simulink model "LAB01P01_simulink"  (R2014a)
settings: Solver=ode45  StartTime=0.0  StopTime=Tstop  MaxStep=1e-5  MinStep=1e-6  RelTol=1e-3
values from neighbouring files (symbols this model uses):
  C1 = 1e-6    (= 1e-06)    [LAB01P01.m]
  C2 = 1e-6    (= 1e-06)    [LAB01P01.m]
  R1 = 1000    [LAB01P01.m]
  R2 = 1000    [LAB01P01.m]
  x0 = [0 0]    [LAB01P01.m]    (also in LAB01P03.m = [0 0]')
settings Model: Creator=S191436  LastModifiedBy=S191436

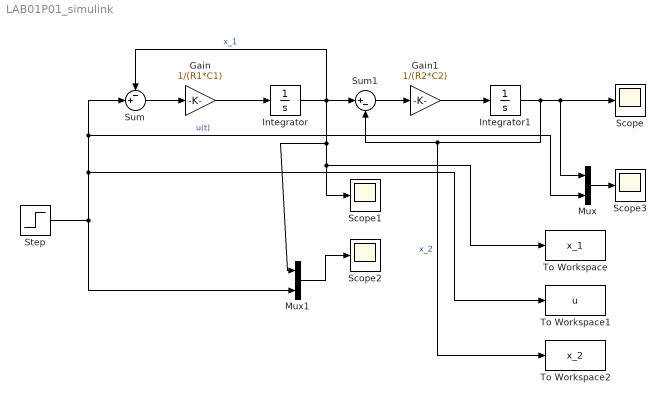
== system LAB01P01_simulink ==
  Gain : Gain  Gain=1/(R1*C1)
  Gain1 : Gain  Gain=1/(R2*C2)
  Integrator : Integrator  InitialCondition=x0(1)
  Integrator1 : Integrator  InitialCondition=x0(2)
  Mux : Mux  Inputs=2
  Mux1 : Mux  Inputs=2
  Scope{,1..3} (4 alike) : Scope
      Scope2 settings: SaveName=ScopeData2
      Scope3 settings: SaveName=ScopeData3
  Step : Step  Time=0  After=2  SampleTime=0
  Sum : Sum  Inputs=-+|
  Sum1 : Sum  Inputs=|+-
  To Workspace : ToWorkspace  VariableName=x_1  SaveFormat=Timeseries  SampleTime=-1
  To Workspace1 : ToWorkspace  VariableName=u  SaveFormat=Timeseries  SampleTime=-1
  To Workspace2 : ToWorkspace  VariableName=x_2  SaveFormat=Timeseries  SampleTime=-1
  wires:
  Gain1/1 -> Integrator1/1
  Sum1/1 -> Gain1/1
  Integrator/1 -> Mux1/1, To Workspace/1, Scope1/1, Sum1/1, Sum/1  "x_1"
  Gain/1 -> Integrator/1
  Sum/1 -> Gain/1
  Integrator1/1 -> Mux/1, Scope/1, To Workspace2/1, Sum1/2  "x_2"
  Mux/1 -> Scope3/1
  Mux1/1 -> Scope2/1
  Step/1 -> To Workspace1/1, Sum/2, Mux/2, Mux1/2  "u(t)"
